simulink model "rpi_camera"  (R2024b)
settings: Solver=FixedStepDiscrete  StartTime=0.0  StopTime=inf  RelTol=1e-3
libraries: LINUX_Library x7, visiontextngfix x3, visionsources x1
settings Model: Creator=petrc  LastModifiedBy=petrc
settings SolverCC: PositivePriorityOrder=on
settings DataIOCC: SaveOutput=off  SignalLogging=off  DSMLogging=off  SaveTime=off  ReturnWorkspaceOutputs=off
settings OptimizationCC: DefaultParameterBehavior=Inlined  EnhancedBackFolding=on  PassReuseOutputArgsAs=Individual arguments  ZeroExternalMemoryAtStartup=off  ZeroInternalMemoryAtStartup=off  MaxStackSize=200000  OptimizeBlockOrder=speed  DifferentSizesBufferReuse=on  OptimizationCustomize=off  EfficientTunableParamExpr=on
settings DebuggingCC: ParameterTunabilityLossMsg=error
settings HardwareCC: ProdBitPerLong=64  ProdLargestAtomicInteger=LongLong  ProdLargestAtomicFloat=Double  ProdLongLongMode=on  ProdHWDeviceType=ARM Compatible->ARM Cortex-A (64-bit)
settings SFSimCC: MATLABDynamicMemAlloc=off  SimTargetLang=C++
settings RTWCC: Description=Real-Time Linux (WSL/Yocto)  SystemTargetFile=rtlinux_ert.tlc  MakeCommand=make_rtw \  GenerateMakefile=off  TemplateMakefile=rtlinux_ert.tmf  Toolchain=GNU GCC Embedded Linux  BuildConfiguration=Faster Runs
settings CodeAppCC: ForceParamTrailComments=on  IgnoreCustomStorageClasses=off  OperatorAnnotations=on  SimulinkDataObjDesc=on  SFDataObjDesc=on  InsertBlockDesc=on
settings STFCustomTargetCC: TargetLibSuffix=.a  TargetLangStandard=C99 (ISO)  MultiwordLength=256  GenerateSampleERTMain=on  CombineOutputUpdateFcns=on  ERTCustomFileBanners=on  SupportContinuousTime=off  SupportNonInlinedSFcns=off  RemoveResetFunc=on  MATLABClassNameForMDSCustomization=Simulink.SoftwareTarget.ERTCustomization  ModelStepFunctionPrototypeControlCompliant=on  SystemTargetFile=rtlinux_ert.tlc
settings ERTTargetCC: TargetLangStandard=C99 (ISO)  GenerateSampleERTMain=on  ParMdlRefBuildCompliant=off  CompOptLevelCompliant=off  ConcurrentExecutionCompliant=off  CPPClassGenCompliant=off  UseToolchainInfoCompliant=off  ERTCustomFileTemplate=LINUX_file_process.tlc

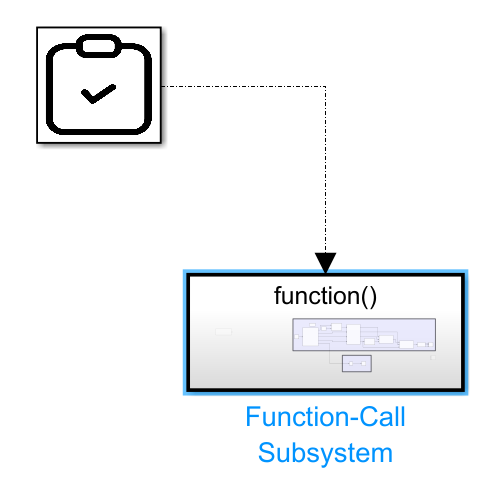
[thumbnail: Simulink's stored preview of the top-level diagram]
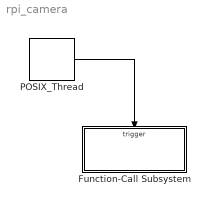
== system rpi_camera ==
  Function-Call Subsystem : Subsystem  TreatAsAtomicUnit=on
  POSIX_Thread : LINUX_Library/POSIX_Thread  TaskName=Camera  TickRes=33  SchedPolicy=SCHED_FIFO  ThreadPriority=99  LockMemory=on  Affinity0=off  Affinity1=on  Affinity2=on  Affinity3=on
      settings: SourceProductName=LINUX Library
  wires:
  POSIX_Thread/1 -> Function-Call Subsystem/Trigger

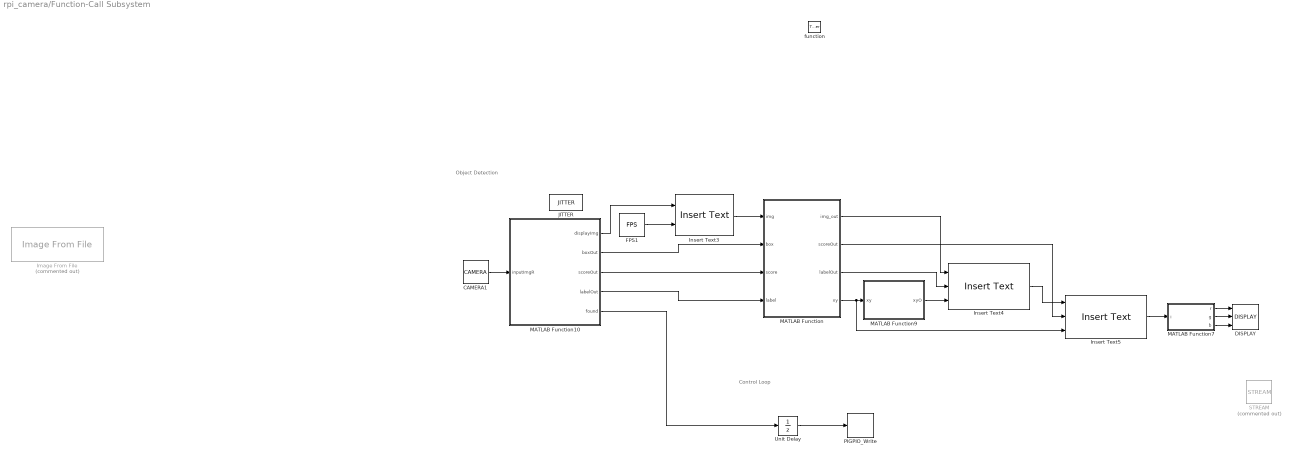
== system rpi_camera/Function-Call Subsystem ==
  note: Control Loop
  note: Object Detection
  function : TriggerPort  TriggerType=function-call  VariantControl=(inherit)
  CAMERA1 : LINUX_Library/CAMERA  device_id=0  width=320  height=320  format=RGB888
      settings: SourceProductName=LINUX Library
  DISPLAY : LINUX_Library/DISPLAY  Width=320  Height=320
      settings: SourceProductName=LINUX Library
  FPS1 : LINUX_Library/FPS
      settings: SourceProductName=LINUX Library
  Image From File : visionsources/Image From File  Tag=vipblks_nd  Commented=on  FileName=C:\Users\petrc\MATLAB\simulink_linux_ert\raspberry\Examples\Inference\plane_resized.png  Ts=inf  imagePorts=One multidimensional signal  OutPortLabels=R|G|B  ImageDataType=Inherit from input image  sdImageDataType=uint(8)  Signed=on  WordLength=16  FractionLengthMode=User-defined  FractionLength=15
  Insert Text3 : visiontextngfix/Insert Text  inputType=Obsolete  theText='FPS: %.2f'  getTextLocFrom=Specify via dialog  textLoc=[1 1]  getTextColorFrom=Specify via dialog  textColor=[255 0 0]  getTextIntensityFrom=Specify via dialog  textIntensity=0  getTextOpacityFrom=Specify via dialog  textOpacity=1.0  dummyVar2=0  dummyVar3=0  dummyVar4=0  imagePorts=One multidimensional signal  isInputTransposed=off  fontFace=LucidaSansRegular  dummyVar1=0  blockFontSize=12  antiAliased=on
  Insert Text4 : visiontextngfix/Insert Text  inputType=Obsolete  theText='%s'  getTextLocFrom=Input port  textLoc=[1 1]  getTextColorFrom=Specify via dialog  textColor=[255,255,0]  getTextIntensityFrom=Specify via dialog  textIntensity=0  getTextOpacityFrom=Specify via dialog  textOpacity=1.0  dummyVar2=0  dummyVar3=0  dummyVar4=0  imagePorts=One multidimensional signal  isInputTransposed=off  fontFace=LucidaSansRegular  dummyVar1=0  blockFontSize=12  antiAliased=off
  Insert Text5 : visiontextngfix/Insert Text  inputType=Obsolete  theText='%.2f'  getTextLocFrom=Input port  textLoc=[1 1]  getTextColorFrom=Specify via dialog  textColor=[255 0 255]  getTextIntensityFrom=Specify via dialog  textIntensity=0  getTextOpacityFrom=Specify via dialog  textOpacity=1.0  dummyVar2=0  dummyVar3=0  dummyVar4=0  imagePorts=One multidimensional signal  isInputTransposed=off  fontFace=LucidaSansRegular  dummyVar1=0  blockFontSize=12  antiAliased=on
  JITTER : LINUX_Library/JITTER  Priority=1  JITTER_NAME=jitter  TICK_RES=33  FRAME_BUFFER=1000000
      settings: SourceProductName=LINUX Library
  MATLAB Function : MATLAB Function  TreatAsAtomicUnit=on
  MATLAB Function10 : MATLAB Function  TreatAsAtomicUnit=on
  MATLAB Function7 : MATLAB Function  TreatAsAtomicUnit=on
  MATLAB Function9 : MATLAB Function  TreatAsAtomicUnit=on
  PIGPIO_Write : LINUX_Library/PIGPIO_Write  Priority=2  io_pin=17
      settings: SourceProductName=LINUX Library
  STREAM : LINUX_Library/STREAM  Commented=on  Width=320  Height=320  FPS=20  Encoder=libx264
      settings: SourceProductName=LINUX Library
  Unit Delay : UnitDelay  SampleTime=-1  HasFrameUpgradeWarning=on
  wires:
  FPS1/1 -> Insert Text3/2
  MATLAB Function10/3(scoreOut) -> MATLAB Function/3(score)
  MATLAB Function10/4(labelOut) -> MATLAB Function/4(label)
  MATLAB Function10/2(boxOut) -> MATLAB Function/2(box)
  Insert Text4/1 -> Insert Text5/1
  MATLAB Function9/1(xyO) -> Insert Text4/3
  MATLAB Function/4(xy) -> Insert Text5/3, MATLAB Function9/1(xy)
  MATLAB Function/3(labelOut) -> Insert Text4/2
  MATLAB Function/2(scoreOut) -> Insert Text5/2
  MATLAB Function/1(img_out) -> Insert Text4/1
  MATLAB Function10/1(displayImg) -> Insert Text3/1
  Insert Text3/1 -> MATLAB Function/1(img)
  Insert Text5/1 -> MATLAB Function7/1(i)
  CAMERA1/1 -> MATLAB Function10/1(inputImgR)
  MATLAB Function7/1(r) -> DISPLAY/1
  MATLAB Function7/2(g) -> DISPLAY/2
  MATLAB Function7/3(b) -> DISPLAY/3
  MATLAB Function10/5(found) -> Unit Delay/1
  Unit Delay/1 -> PIGPIO_Write/1

== matlab function rpi_camera/Function-Call Subsystem/MATLAB Function ==
  data: img input; img_out output; box input; score input; label input; scoreOut output; labelOut output; xy output
function [img_out, scoreOut, labelOut, xy]  = DrawBoxes(img, box, score, label)

img_out = img;
[H, W, ~] = size(img_out);
lineWidth = 2;

% fprintf("%f\r\n", score);

if score > 60
    x = int32(box(2) * W);
    y = int32(box(1) * H);
    x2 = int32(box(4) * W);
    y2 = int32(box(3) * H);

    w = x2-x;
    h = y2-y;

    scoreOut = score;
    labelOut = label;
    xy = [x, y - 20];
    % fprintf("%d %d %d %d\r\n", x, y, w, h);
    
    for l = 0:lineWidth-1
        yt = y + l;
        yb = y + h - l;
        xl = x + l;
        xr = x + w - l;
    
        if yt <= H
            img_out(yt, x:x+w, 1) = uint8(255);
            img_out(yt, x:x+w, 2) = uint8(0);
            img_out(yt, x:x+w, 3) = uint8(0);
        end
        if yb <= H
            img_out(yb, x:x+w, 1) = uint8(255);
            img_out(yb, x:x+w, 2) = uint8(0);
            img_out(yb, x:x+w, 3) = uint8(0);
        end
        if xl <= W
            img_out(y:y+h, xl, 1) = uint8(255);
            img_out(y:y+h, xl, 2) = uint8(0);
            img_out(y:y+h, xl, 3) = uint8(0);
        end
        if xr <= W
            img_out(y:y+h, xr, 1) = uint8(255);
            img_out(y:y+h, xr, 2) = uint8(0);
            img_out(y:y+h, xr, 3) = uint8(0);
        end
    end
else
    scoreOut = score;
    labelOut = label;
    xy = [int32(1000), int32(1000)];
end

end

== matlab function rpi_camera/Function-Call Subsystem/MATLAB Function7 ==
  data: i input; r output; g output; b output
function [r,g,b] = ImageToRGB(i)
%#codegen
r =i(:,:,1);
g =i(:,:,2);
b =i(:,:,3);
end

== matlab function rpi_camera/Function-Call Subsystem/MATLAB Function10 ==
  data: displayImg output; inputImgR input; boxOut output; scoreOut output; labelOut output; found output
function [displayImg, boxOut, scoreOut, labelOut, found] = TFlitePredict(inputImgR)
%#codegen

persistent net;
persistent cocoLabels;

if isempty(net)
    net = loadTFLiteModel("ssd_mobilenet.tflite");

    % Replace your cocoLabels with this structure (shortened for brevity)
    cocoLabels = {'person', 'bicycle', 'car', 'motorcycle', 'airplane', 'bus', 'train', 'truck', 'boat', 'traffic light', ...
        'fire hydrant', 'street sign', 'stop sign', 'parking meter', 'bench', 'bird', 'cat', 'dog', 'horse', 'sheep', ...
        'cow', 'elephant', 'bear', 'zebra', 'giraffe', 'hat', 'backpack', 'umbrella', 'shoe', 'eye glasses', ...
        'handbag', 'tie', 'suitcase', 'frisbee', 'skis', 'snowboard', 'sports ball', 'kite', 'baseball bat', 'baseball glove', ...
        'skateboard', 'surfboard', 'tennis racket', 'bottle', 'plate', 'wine glass', 'cup', 'fork', 'knife', 'spoon', ...
        'bowl', 'banana', 'apple', 'sandwich', 'orange', 'broccoli', 'carrot', 'hot dog', 'pizza', 'donut', ...
        'cake', 'chair', 'couch', 'potted plant', 'bed', 'mirror', 'dining table', 'window', 'desk', 'toilet', ...
        'door', 'tv', 'laptop', 'mouse', 'remote', 'keyboard', 'cell phone', 'microwave', 'oven', 'toaster', ...
        'sink', 'refrigerator', 'blender', 'book', 'clock', 'vase', 'scissors', 'teddy bear', 'hair drier', 'toothbrush', 'hair brush'};
end


raw3D = reshape(inputImgR, [3, 320, 320]);
imgRestored = permute(raw3D, [3, 2, 1]);
displayImg = imgRestored;
imgRGB = imgRestored(:, :, [3 2 1]);

[boxes, labels, scores, ~] = predict(net, imgRGB, "EnableINT8InferenceOnWindows", true);

[maxScore, maxIdx] = max(scores);

scoreOut = maxScore * 100;
boxOut = boxes(maxIdx, :);
labelNum = labels(maxIdx) + 1;
if labelNum >= 1 && labelNum <= numel(cocoLabels)
    name = cocoLabels{labelNum};
else
    name = 'unknown';
end

labelOut = zeros(1,20,'uint8');
len = min(length(name), 20);
labelOut(1:len) = uint8(name(1:len));

if scoreOut > 60
    found = 1;
else
    found = 0;
end


end

== matlab function rpi_camera/Function-Call Subsystem/MATLAB Function9 ==
  data: xy input; xyO output
function xyO  = fcn(xy)

xyO = [xy(1) + 40, xy(2)];
